simulink model "sensorMCU"  (Simulink 6.6)
settings: Solver=FixedStepDiscrete  StartTime=0.0  StopTime=10.0  FixedStep=0.01  RelTol=1e-3
InitFcn:
  | mcuInit
values from neighbouring files (symbols this model uses):
  gxGainrad = gxGain*pi/180    [mcuInit.m]
  gyGainrad = gyGain*pi/180    [mcuInit.m]
  gzGainrad = gzGain*pi/180    [mcuInit.m]
  T = 0.01    [initGPS.m]    (also in mcuInit.m)
undefined symbols (not defined in the file or in its folder): AccelParam, floatToBytes, gaind, gpsInit, gpsParse, gpsRead, gpsSeparate, gyTGain, hil_getEuler, hil_getGPSRead, hil_getRates, hil_getRawRead, hil_getVned, hil_getXYZ, hilRead, logData, loggerInit, MagParam, mzTGain, polesd, protParseDecode, protParserInit, shortToBytes, spiMasterInit, spiSend, stTGain, tmeanMz, tmeanSt, tmeanVl, u1, uartInit, uShortToBytes, vlTGain, y1, zerosd
libraries: dsPICdrivers x72, simulink x6, dspswit3 x1, dspsigops x1, xpclib x1, aerolibconvert2 x1
(part 2 of 3)

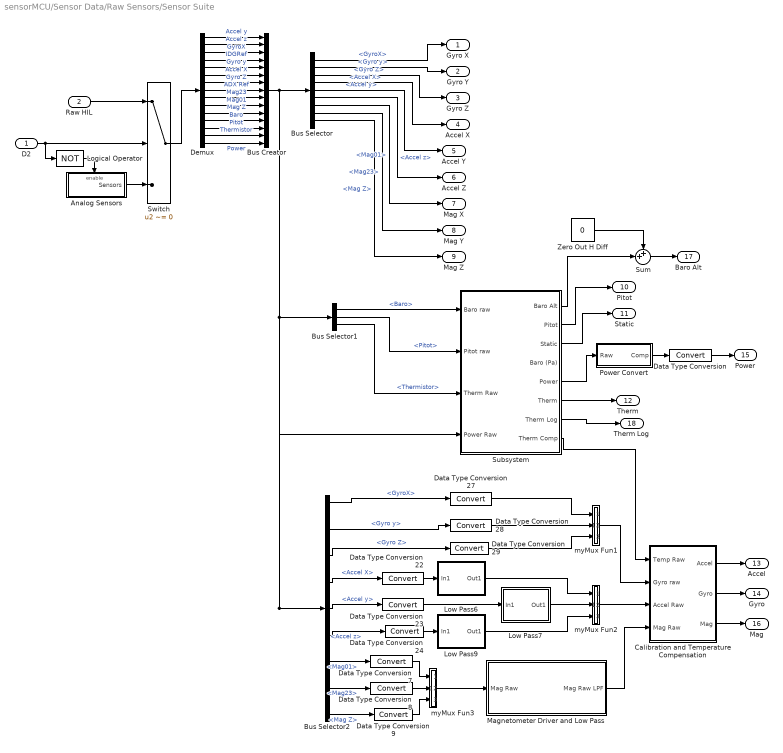
== system sensorMCU/Sensor Data/Raw Sensors/Sensor Suite ==
  D2 : Inport
  Raw HIL : Inport  Port=2
  Analog Sensors : Subsystem
  Bus Creator : BusCreator  Inputs=15
  Bus Selector : BusSelector  OutputSignals=GyroX,Gyro y,Gyro Z,Accel X,Accel y,Accel z,Mag01,Mag23,Mag Z
  Bus Selector1 : BusSelector  OutputSignals=Baro,Pitot,Thermistor
  Bus Selector2 : BusSelector  OutputSignals=GyroX,Gyro y,Gyro Z,Accel X,Accel y,Accel z,Mag01,Mag23,Mag Z
  Calibration and Temperature Compensation : Subsystem
  Data Type Conversion : DataTypeConversion  OutDataTypeMode=uint16
  Data Type Conversion{7..9,22..24,27..29} (9 alike) : DataTypeConversion  OutDataTypeMode=double
  Demux : Demux  Outputs=15
  Logical Operator : Logic  Operator=NOT  AllPortsSameDT=off  OutDataTypeMode=Boolean
  Low Pass6 : Subsystem  mask(DiscretizedZeroPole){Zeros=[], Poles=[-150], Gain=150, AbsTol=auto, SampleTime=T, method=tustin, Wc=1}
      mask prompts: Zeros "Zeros (enter in s-main:)"; Poles "Poles (enter in s-domain:)"; Gain "Gain (enter in s-domain:)"; AbsTol "Absolute tolerance:"; SampleTime "Sample time:"; Wc "Critical Frequency (Hz):"
      mask help: Continuous mask uses c2d to transform parameters onto the Discrete Zero-Pole block inside.
      mask init:
      | st=SampleTime;
      | if length(st)>1
      |     st=SampleTime(1);
      | end
      | if(st>0)
      |     [zerosd,polesd,gaind] = sldiscutil('disczpk', {st,method,Wc,Zeros,Poles,Gain});
      | end	
      | s = get_param(gcb,'maskvalues');
      | zeross = s{1};
      | poless = s{2};
      | gainss = s{3};
      | %zerosc = eval(zeross);
      | %polesc = eval(poless);
      | %gainsc = eval(gainss);
      | sldiscutil('initzpkmask', st);
      | if(st==0)
      | set_param([gcb '/Zero Pole'], 'AbsoluteTolerance', AbsTol);
      | end
      mask StyleString: edit,edit,edit,edit,edit,popup(zoh|foh|tustin|prewarp|matched),edit
      mask CallbackString: |||||hidecrit|
      mask Display:
      | droots(zeross,poless,gainss)
      | text( 0.5, 1.0, method, 'verticalAlignment','top')
  Low Pass7 : Subsystem  mask(DiscretizedZeroPole){Zeros=[], Poles=[-150], Gain=150, AbsTol=auto, SampleTime=T, method=tustin, Wc=1}
      mask prompts: Zeros "Zeros (enter in s-main:)"; Poles "Poles (enter in s-domain:)"; Gain "Gain (enter in s-domain:)"; AbsTol "Absolute tolerance:"; SampleTime "Sample time:"; Wc "Critical Frequency (Hz):"
      mask help: Continuous mask uses c2d to transform parameters onto the Discrete Zero-Pole block inside.
      mask init: same as sensorMCU/Sensor Data/Raw Sensors/Sensor Suite/Low Pass6
      mask StyleString: edit,edit,edit,edit,edit,popup(zoh|foh|tustin|prewarp|matched),edit
      mask CallbackString: |||||hidecrit|
      mask Display:
      | droots(zeross,poless,gainss)
      | text( 0.5, 1.0, method, 'verticalAlignment','top')
  Low Pass9 : Subsystem  mask(DiscretizedZeroPole){Zeros=[], Poles=[-150], Gain=150, AbsTol=auto, SampleTime=T, method=tustin, Wc=1}
      mask prompts: Zeros "Zeros (enter in s-main:)"; Poles "Poles (enter in s-domain:)"; Gain "Gain (enter in s-domain:)"; AbsTol "Absolute tolerance:"; SampleTime "Sample time:"; Wc "Critical Frequency (Hz):"
      mask help: Continuous mask uses c2d to transform parameters onto the Discrete Zero-Pole block inside.
      mask init: same as sensorMCU/Sensor Data/Raw Sensors/Sensor Suite/Low Pass6
      mask StyleString: edit,edit,edit,edit,edit,popup(zoh|foh|tustin|prewarp|matched),edit
      mask CallbackString: |||||hidecrit|
      mask Display:
      | droots(zeross,poless,gainss)
      | text( 0.5, 1.0, method, 'verticalAlignment','top')
  Magnetometer Driver and Low Pass : Subsystem
  Power Convert : Subsystem  mask{bias=0.02946, gains=0.003226}
      mask prompts: bias "Initial Bias"; gains "Initial Gains"
      mask help: Convert Analog readings to units
  Subsystem : Subsystem
  Sum : Sum  Inputs=++|
  Switch : Switch  Criteria=u2 ~= 0  SampleTime=0.01
  Zero Out H Diff : Constant  Value=0
  myMux Fun1 : Stateflow chart
  myMux Fun2 : Stateflow chart
  myMux Fun3 : Stateflow chart
  Gyro X : Outport
  Gyro Y : Outport  Port=2
  Gyro Z : Outport  Port=3
  Accel X : Outport  Port=4
  Accel Y : Outport  Port=5
  Accel Z : Outport  Port=6
  Mag X : Outport  Port=7
  Mag Y : Outport  Port=8
  Mag Z : Outport  Port=9
  Pitot : Outport  Port=10
  Static : Outport  Port=11
  Therm : Outport  Port=12
  Accel : Outport  Port=13
  Gyro : Outport  Port=14
  Power : Outport  Port=15
  Mag : Outport  Port=16
  Baro Alt : Outport  Port=17
  Therm Log : Outport  Port=18
  wires:
  Demux/1 -> Bus Creator/1  "Accel y"
  Demux/2 -> Bus Creator/2  "Accel z"
  Demux/3 -> Bus Creator/3  "GyroX"
  Demux/4 -> Bus Creator/4  "IDGRef"
  Demux/5 -> Bus Creator/5  "Gyro y"
  Demux/6 -> Bus Creator/6  "Accel X"
  Demux/7 -> Bus Creator/7  "Gyro Z"
  Demux/8 -> Bus Creator/8  "ADX Ref"
  Demux/9 -> Bus Creator/9  "Mag23"
  Demux/10 -> Bus Creator/10  "Mag01"
  Demux/11 -> Bus Creator/11  "Mag Z"
  Demux/12 -> Bus Creator/12  "Baro"
  Demux/13 -> Bus Creator/13  "Pitot"
  Demux/14 -> Bus Creator/14  "Thermistor"
  Demux/15 -> Bus Creator/15  "Power"
  Bus Creator/1 -> Bus Selector/1, Bus Selector1/1, Bus Selector2/1, Subsystem/4(Power Raw)
  Bus Selector1/1 -> Subsystem/1(Baro raw)  "<Baro>"
  Data Type Conversion27/1 -> myMux Fun1/1(u1)
  Data Type Conversion28/1 -> myMux Fun1/2(u2)
  Data Type Conversion29/1 -> myMux Fun1/3(u3)
  Low Pass6/1(Out1) -> myMux Fun2/1(u1)
  Low Pass7/1(Out1) -> myMux Fun2/2(u2)
  Data Type Conversion22/1 -> Low Pass6/1(In1)
  Data Type Conversion23/1 -> Low Pass7/1(In1)
  Data Type Conversion24/1 -> Low Pass9/1(In1)
  Low Pass9/1(Out1) -> myMux Fun2/3(u3)
  Bus Selector/1 -> Gyro X/1  "<GyroX>"
  Bus Selector/2 -> Gyro Y/1  "<Gyro y>"
  Bus Selector/3 -> Gyro Z/1  "<Gyro Z>"
  Bus Selector/4 -> Accel X/1  "<Accel X>"
  Bus Selector/5 -> Accel Y/1  "<Accel y>"
  Bus Selector/6 -> Accel Z/1  "<Accel z>"
  Bus Selector/7 -> Mag X/1  "<Mag01>"
  Bus Selector/8 -> Mag Y/1  "<Mag23>"
  Bus Selector/9 -> Mag Z/1  "<Mag Z>"
  Bus Selector2/1 -> Data Type Conversion27/1  "<GyroX>"
  Bus Selector2/2 -> Data Type Conversion28/1  "<Gyro y>"
  Bus Selector2/3 -> Data Type Conversion29/1  "<Gyro Z>"
  Bus Selector2/4 -> Data Type Conversion22/1  "<Accel X>"
  Bus Selector2/5 -> Data Type Conversion23/1  "<Accel y>"
  Bus Selector2/6 -> Data Type Conversion24/1  "<Accel z>"
  myMux Fun1/1(y) -> Calibration and Temperature Compensation/2(Gyro raw)
  myMux Fun2/1(y) -> Calibration and Temperature Compensation/3(Accel Raw)
  Bus Selector1/2 -> Subsystem/2(Pitot raw)  "<Pitot>"
  Bus Selector1/3 -> Subsystem/3(Therm Raw)  "<Thermistor>"
  Switch/1 -> Demux/1
  D2/1 -> Switch/2, Logical Operator/1
  Analog Sensors/1(Sensors) -> Switch/3
  Logical Operator/1 -> Analog Sensors/Enable
  Raw HIL/1 -> Switch/1
  Data Type Conversion7/1 -> myMux Fun3/1(u1)
  Data Type Conversion8/1 -> myMux Fun3/2(u2)
  Data Type Conversion9/1 -> myMux Fun3/3(u3)
  myMux Fun3/1(y) -> Magnetometer Driver and Low Pass/1(Mag Raw)
  Bus Selector2/7 -> Data Type Conversion7/1  "<Mag01>"
  Bus Selector2/8 -> Data Type Conversion8/1  "<Mag23>"
  Bus Selector2/9 -> Data Type Conversion9/1  "<Mag Z>"
  Calibration and Temperature Compensation/3(Mag) -> Mag/1
  Calibration and Temperature Compensation/1(Accel) -> Accel/1
  Calibration and Temperature Compensation/2(Gyro) -> Gyro/1
  Magnetometer Driver and Low Pass/1(Mag Raw LPF) -> Calibration and Temperature Compensation/4(Mag Raw)
  Subsystem/8(Therm Comp) -> Calibration and Temperature Compensation/1(Temp Raw)
  Subsystem/2(Pitot) -> Pitot/1
  Subsystem/3(Static) -> Static/1
  Subsystem/5(Power) -> Power Convert/1(Raw)
  Subsystem/6(Therm) -> Therm/1
  Subsystem/7(Therm Log) -> Therm Log/1
  Power Convert/1(Comp) -> Data Type Conversion/1
  Data Type Conversion/1 -> Power/1
  Sum/1 -> Baro Alt/1
  Subsystem/1(Baro Alt) -> Sum/2
  Zero Out H Diff/1 -> Sum/1

== system sensorMCU/Position-Attitude Filter/GPS parser/GPS Update/Detect Change ==
  Data : Inport
  Abs1 : Abs
  Difference1 : simulink/Discrete/Difference  SystemSampleTime=-1  ICPrevInput=0.0  OutDataType=sfix(16)  OutScaling=2^-10  DoSatur=off
  Saturation1 : Saturate  UpperLimit=1  LowerLimit=0
  change? : Outport
  wires:
  Difference1/1 -> Abs1/1
  Abs1/1 -> Saturation1/1
  Data/1 -> Difference1/1
  Saturation1/1 -> change?/1

== system sensorMCU/Position-Attitude Filter/GPS parser/GPS Update/Detect Change1 ==
  Data : Inport
  Abs1 : Abs
  Difference1 : simulink/Discrete/Difference  SystemSampleTime=-1  ICPrevInput=0.0  OutDataType=sfix(16)  OutScaling=2^-10  DoSatur=off
  Saturation1 : Saturate  UpperLimit=1  LowerLimit=0
  change? : Outport
  wires:
  Saturation1/1 -> change?/1
  Data/1 -> Difference1/1
  Abs1/1 -> Saturation1/1
  Difference1/1 -> Abs1/1

== system sensorMCU/Position-Attitude Filter/GPS parser/GPS Update/Detect Change2 ==
  Data : Inport
  Abs1 : Abs
  Difference1 : simulink/Discrete/Difference  SystemSampleTime=-1  ICPrevInput=0.0  OutDataType=sfix(16)  OutScaling=2^-10  DoSatur=off
  Saturation1 : Saturate  UpperLimit=1  LowerLimit=0
  change? : Outport
  wires:
  Difference1/1 -> Abs1/1
  Abs1/1 -> Saturation1/1
  Data/1 -> Difference1/1
  Saturation1/1 -> change?/1

== system sensorMCU/Position-Attitude Filter/GPS parser/Geod2LTP2/ECEF2LTP (UEN) ==
  ECEF coordinates : Inport
  "Long, Lat" : Inport  Port=2
  Deg2R : Gain  Gain=pi/180  SaturateOnIntegerOverflow=on
  Demux3 : Demux  Outputs=2
  From Body to Universal1 : Subsystem
  Product1 : Product  Multiplication=Matrix(*)  SaturateOnIntegerOverflow=on  InputSameDT=on
  Out : Outport
  wires:
  "Long, Lat"/1 -> Deg2R/1
  Product1/1 -> Out/1
  Demux3/2 -> From Body to Universal1/2(lat)
  Demux3/1 -> From Body to Universal1/1(long)
  Deg2R/1 -> Demux3/1
  ECEF coordinates/1 -> Product1/2
  From Body to Universal1/1(DCM) -> Product1/1

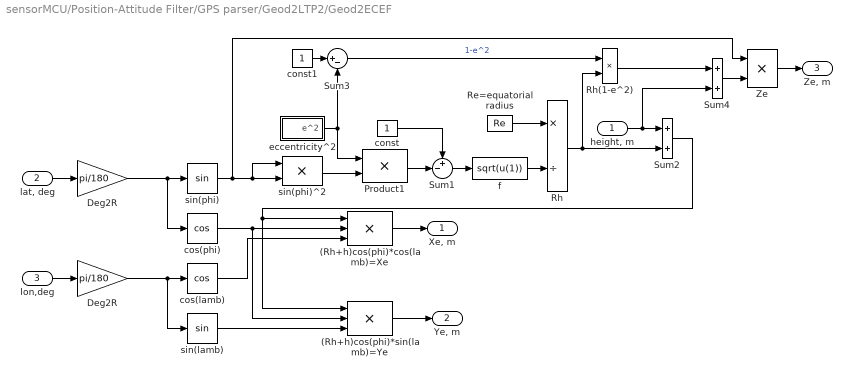
== system sensorMCU/Position-Attitude Filter/GPS parser/Geod2LTP2/Geod2ECEF ==
  "height, m" : Inport
  "lat, deg" : Inport  Port=2
  lon,deg : Inport  Port=3
  (Rh+h)cos(phi)*cos(lamb)=Xe : Product  Inputs=3  SaturateOnIntegerOverflow=on  InputSameDT=on
  (Rh+h)cos(phi)*sin(lamb)=Ye : Product  Inputs=3  SaturateOnIntegerOverflow=on  InputSameDT=on
  Deg2R : Gain  Gain=pi/180  SaturateOnIntegerOverflow=on
  "Deg2R " : Gain  Gain=pi/180  SaturateOnIntegerOverflow=on
  Product1 : Product  SaturateOnIntegerOverflow=on  InputSameDT=on
  Re=equatorial radius : Constant  Value=Re
  Rh : Product  Inputs=*/  SaturateOnIntegerOverflow=on  InputSameDT=on
  Rh(1-e^2) : Product  SaturateOnIntegerOverflow=on  InputSameDT=on
  Sum1 : Sum  Inputs=+-|  SaturateOnIntegerOverflow=on  InputSameDT=on
  Sum2 : Sum  SaturateOnIntegerOverflow=on  InputSameDT=on
      settings: AttributesFormatString=Rh+h
  Sum3 : Sum  Inputs=|+-  SaturateOnIntegerOverflow=on  InputSameDT=on
  Sum4 : Sum  SaturateOnIntegerOverflow=on  InputSameDT=on
      settings: AttributesFormatString=(1-e^2)Rh+h
  Ze : Product  SaturateOnIntegerOverflow=on  InputSameDT=on
  const : Constant
  const1 : Constant
  cos(lamb) : Trigonometry  Operator=cos
  cos(phi) : Trigonometry  Operator=cos
  eccentricity^2 : Subsystem
  f : Fcn  Expr=sqrt(u(1))
  sin(lamb) : Trigonometry
  sin(phi) : Trigonometry
  sin(phi)^2 : Product  SaturateOnIntegerOverflow=on  InputSameDT=on
  "Xe, m " : Outport
  "Ye, m " : Outport  Port=2
  "Ze, m " : Outport  Port=3
  wires:
  "lat, deg"/1 -> Deg2R/1
  sin(phi)/1 -> sin(phi)^2/1, sin(phi)^2/2, Ze/1
  f/1 -> Rh/2
  Re=equatorial radius/1 -> Rh/1
  Rh/1 -> Sum2/2, Rh(1-e^2)/2
  Product1/1 -> Sum1/2
  Sum1/1 -> f/1
  const/1 -> Sum1/1
  "height, m"/1 -> Sum4/2, Sum2/1
  eccentricity^2/1(e^2) -> Product1/1, Sum3/2
  sin(phi)^2/1 -> Product1/2
  const1/1 -> Sum3/1
  Sum3/1 -> Rh(1-e^2)/1  "1-e^2"
  Rh(1-e^2)/1 -> Sum4/1
  Sum4/1 -> Ze/2
  lon,deg/1 -> "Deg2R "/1
  cos(phi)/1 -> (Rh+h)cos(phi)*cos(lamb)=Xe/2, (Rh+h)cos(phi)*sin(lamb)=Ye/2
  cos(lamb)/1 -> (Rh+h)cos(phi)*cos(lamb)=Xe/3
  sin(lamb)/1 -> (Rh+h)cos(phi)*sin(lamb)=Ye/3
  Ze/1 -> "Ze, m "/1
  Deg2R/1 -> cos(phi)/1, sin(phi)/1
  "Deg2R "/1 -> cos(lamb)/1, sin(lamb)/1
  Sum2/1 -> (Rh+h)cos(phi)*sin(lamb)=Ye/1, (Rh+h)cos(phi)*cos(lamb)=Xe/1
  (Rh+h)cos(phi)*cos(lamb)=Xe/1 -> "Xe, m "/1
  (Rh+h)cos(phi)*sin(lamb)=Ye/1 -> "Ye, m "/1

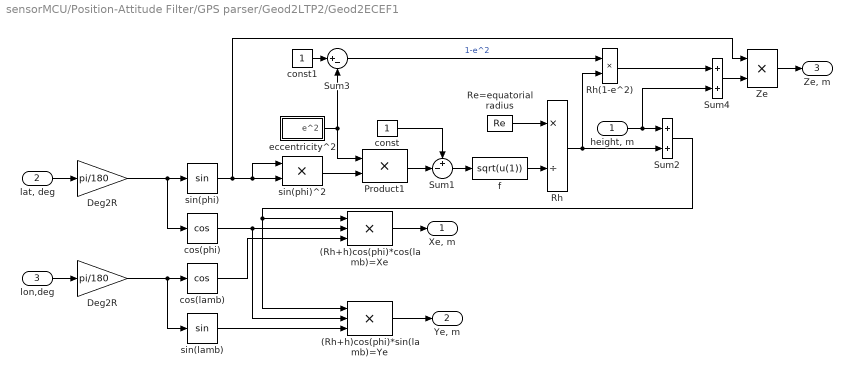
== system sensorMCU/Position-Attitude Filter/GPS parser/Geod2LTP2/Geod2ECEF1 ==
  "height, m" : Inport
  "lat, deg" : Inport  Port=2
  lon,deg : Inport  Port=3
  (Rh+h)cos(phi)*cos(lamb)=Xe : Product  Inputs=3  SaturateOnIntegerOverflow=on  InputSameDT=on
  (Rh+h)cos(phi)*sin(lamb)=Ye : Product  Inputs=3  SaturateOnIntegerOverflow=on  InputSameDT=on
  Deg2R : Gain  Gain=pi/180  SaturateOnIntegerOverflow=on
  "Deg2R " : Gain  Gain=pi/180  SaturateOnIntegerOverflow=on
  Product1 : Product  SaturateOnIntegerOverflow=on  InputSameDT=on
  Re=equatorial radius : Constant  Value=Re
  Rh : Product  Inputs=*/  SaturateOnIntegerOverflow=on  InputSameDT=on
  Rh(1-e^2) : Product  SaturateOnIntegerOverflow=on  InputSameDT=on
  Sum1 : Sum  Inputs=+-|  SaturateOnIntegerOverflow=on  InputSameDT=on
  Sum2 : Sum  SaturateOnIntegerOverflow=on  InputSameDT=on
      settings: AttributesFormatString=Rh+h
  Sum3 : Sum  Inputs=|+-  SaturateOnIntegerOverflow=on  InputSameDT=on
  Sum4 : Sum  SaturateOnIntegerOverflow=on  InputSameDT=on
      settings: AttributesFormatString=(1-e^2)Rh+h
  Ze : Product  SaturateOnIntegerOverflow=on  InputSameDT=on
  const : Constant
  const1 : Constant
  cos(lamb) : Trigonometry  Operator=cos
  cos(phi) : Trigonometry  Operator=cos
  eccentricity^2 : Subsystem
  f : Fcn  Expr=sqrt(u(1))
  sin(lamb) : Trigonometry
  sin(phi) : Trigonometry
  sin(phi)^2 : Product  SaturateOnIntegerOverflow=on  InputSameDT=on
  "Xe, m " : Outport
  "Ye, m " : Outport  Port=2
  "Ze, m " : Outport  Port=3
  wires:
  (Rh+h)cos(phi)*sin(lamb)=Ye/1 -> "Ye, m "/1
  (Rh+h)cos(phi)*cos(lamb)=Xe/1 -> "Xe, m "/1
  Sum2/1 -> (Rh+h)cos(phi)*cos(lamb)=Xe/1, (Rh+h)cos(phi)*sin(lamb)=Ye/1
  "Deg2R "/1 -> sin(lamb)/1, cos(lamb)/1
  Deg2R/1 -> sin(phi)/1, cos(phi)/1
  Ze/1 -> "Ze, m "/1
  sin(lamb)/1 -> (Rh+h)cos(phi)*sin(lamb)=Ye/3
  cos(lamb)/1 -> (Rh+h)cos(phi)*cos(lamb)=Xe/3
  cos(phi)/1 -> (Rh+h)cos(phi)*sin(lamb)=Ye/2, (Rh+h)cos(phi)*cos(lamb)=Xe/2
  lon,deg/1 -> "Deg2R "/1
  Sum4/1 -> Ze/2
  Rh(1-e^2)/1 -> Sum4/1
  Sum3/1 -> Rh(1-e^2)/1  "1-e^2"
  const1/1 -> Sum3/1
  sin(phi)^2/1 -> Product1/2
  eccentricity^2/1(e^2) -> Sum3/2, Product1/1
  "height, m"/1 -> Sum2/1, Sum4/2
  const/1 -> Sum1/1
  Sum1/1 -> f/1
  Product1/1 -> Sum1/2
  Rh/1 -> Rh(1-e^2)/2, Sum2/2
  Re=equatorial radius/1 -> Rh/1
  f/1 -> Rh/2
  sin(phi)/1 -> Ze/1, sin(phi)^2/2, sin(phi)^2/1
  "lat, deg"/1 -> Deg2R/1

== system sensorMCU/Sensor Data/Raw Sensors/Sensor Suite/Analog Sensors ==
  Enable : EnablePort
  ADC Input : dsPICdrivers/Peripheral I//O/ADC Input  Tag=dsPIC_ADC  Priority=5  ADC_TYPE=12 bits  ADC_MODE=Continuous sampling & get last channel value  NbrSampleStep=1  VoltRefpopup="AVdd  -  AVss"  OutFormatBitspopup=0000 dddd dddd dddd : Integer  InterruptPriority=6  ANCHANNELS=[0 1 3 4 5 6 7 8 9 10 11 12 13 15 16]  MaxName=ANmax = 4096  Rin=1e2  ADCS=53  SAMC=1  Temperature=25  DMAChannel=1  SampleTime=.01  Status="OK  |  Tsmp=6.750e-007 |  T/Channel=1.012e-005 |  Tall=1.519e-004"
  Mux : Mux  Inputs=15
  Sensors : Outport
  wires:
  ADC Input/1 -> Mux/1
  ADC Input/2 -> Mux/2
  ADC Input/3 -> Mux/3
  ADC Input/4 -> Mux/4
  ADC Input/5 -> Mux/5
  ADC Input/6 -> Mux/6
  ADC Input/7 -> Mux/7
  ADC Input/8 -> Mux/8
  ADC Input/9 -> Mux/9
  ADC Input/10 -> Mux/10
  ADC Input/11 -> Mux/11
  ADC Input/12 -> Mux/12
  ADC Input/13 -> Mux/13
  ADC Input/14 -> Mux/14
  ADC Input/15 -> Mux/15
  Mux/1 -> Sensors/1

== system sensorMCU/Sensor Data/Raw Sensors/Sensor Suite/Calibration and Temperature Compensation ==
  Temp Raw : Inport
  Gyro raw : Inport  Port=2
  Accel Raw : Inport  Port=3
  Mag Raw : Inport  Port=4
  AccelConvert : Subsystem  mask{bias=[AccelParam.xo AccelParam.yo AccelParam.zo], gains=[-AccelParam.a AccelParam.b  -AccelParam.c]}
      mask prompts: bias "Initial Bias"; gains "Initial Gains"
      mask help: Convert Analog readings to units
  Divide : Product  OutScaling=2^-10
  Enables/Disables the Computation of  initial Biases and Temps : Stateflow chart
  Gyro Gains : Constant  Value=[-gxGainrad gyGainrad gzGainrad]
  Gyro Temp  Compensation : Subsystem  mask{alpha=[0 gyTGain 0]}
      mask prompts: alpha "Gyro Tempearature Coeficientt"
      mask help: Temperature Compensate Gyro Measurement
  Initial Bias and Temp : Subsystem  TreatAsAtomicUnit=on
  Mag Convert : Subsystem  mask{bias=[MagParam.xo MagParam.yo MagParam.zo], gains=[MagParam.a MagParam.b  MagParam.c]}
      mask prompts: bias "Initial Bias"; gains "Initial Gains"
      mask help: Convert Analog readings to units
  Mag Temp  Compensation : Subsystem  mask{alpha=[0 0 mzTGain], tempMean=[0 0 tmeanMz]}
      mask prompts: alpha "Tempearature Coeficientt"; tempMean "Calibration Mean Temperature"
      mask help: Temperature Compensate Gyro Measurement
  Accel : Outport
  Gyro : Outport  Port=2
  Mag : Outport  Port=3
  wires:
  AccelConvert/1(Comp) -> Accel/1
  Accel Raw/1 -> AccelConvert/1(Raw)
  Enables/Disables the Computation of  initial Biases and Temps/1(tOut) -> Initial Bias and Temp/Enable
  Temp Raw/1 -> Initial Bias and Temp/1(Temp Raw), Gyro Temp  Compensation/4(Temp Raw), Mag Temp  Compensation/1(Temp Raw)
  Gyro raw/1 -> Initial Bias and Temp/2(Gyro Raw), Gyro Temp  Compensation/3(Raw)
  Initial Bias and Temp/2(Gyro Ini Bias) -> Gyro Temp  Compensation/2(Bias Ini)
  Initial Bias and Temp/1(Temp Ini) -> Gyro Temp  Compensation/1(Temp Ini)
  Gyro Temp  Compensation/1(Comp) -> Divide/1
  Gyro Gains/1 -> Divide/2
  Divide/1 -> Gyro/1
  Mag Raw/1 -> Mag Temp  Compensation/2(Raw)
  Mag Convert/1(Comp) -> Mag/1
  Mag Temp  Compensation/1(Comp) -> Mag Convert/1(Raw)

== system sensorMCU/Sensor Data/Raw Sensors/Sensor Suite/Low Pass6 ==
  In1 : Inport
  Discrete Zero-Pole : DiscreteZeroPole  Zeros=zerosd  Poles=polesd  Gain=gaind  SampleTime=SampleTime
  Out1 : Outport
  wires:
  In1/1 -> Discrete Zero-Pole/1
  Discrete Zero-Pole/1 -> Out1/1

== system sensorMCU/Sensor Data/Raw Sensors/Sensor Suite/Low Pass7 ==
  In1 : Inport
  Discrete Zero-Pole : DiscreteZeroPole  Zeros=zerosd  Poles=polesd  Gain=gaind  SampleTime=SampleTime
  Out1 : Outport
  wires:
  Discrete Zero-Pole/1 -> Out1/1
  In1/1 -> Discrete Zero-Pole/1

== system sensorMCU/Sensor Data/Raw Sensors/Sensor Suite/Low Pass9 ==
  In1 : Inport
  Discrete Zero-Pole : DiscreteZeroPole  Zeros=zerosd  Poles=polesd  Gain=gaind  SampleTime=SampleTime
  Out1 : Outport
  wires:
  Discrete Zero-Pole/1 -> Out1/1
  In1/1 -> Discrete Zero-Pole/1

== system sensorMCU/Sensor Data/Raw Sensors/Sensor Suite/Magnetometer Driver and Low Pass ==
  Mag Raw : Inport
  Demux1 : Demux  Outputs=3
  Low Pass3 : Subsystem  mask(DiscretizedZeroPole){Zeros=[], Poles=[-150], Gain=150, AbsTol=auto, SampleTime=T, method=tustin, Wc=1}
      mask prompts: Zeros "Zeros (enter in s-main:)"; Poles "Poles (enter in s-domain:)"; Gain "Gain (enter in s-domain:)"; AbsTol "Absolute tolerance:"; SampleTime "Sample time:"; Wc "Critical Frequency (Hz):"
      mask help: Continuous mask uses c2d to transform parameters onto the Discrete Zero-Pole block inside.
      mask init: same as sensorMCU/Sensor Data/Raw Sensors/Sensor Suite/Low Pass6
      mask StyleString: edit,edit,edit,edit,edit,popup(zoh|foh|tustin|prewarp|matched),edit
      mask CallbackString: |||||hidecrit|
      mask Display:
      | droots(zeross,poless,gainss)
      | text( 0.5, 1.0, method, 'verticalAlignment','top')
  Low Pass4 : Subsystem  mask(DiscretizedZeroPole){Zeros=[], Poles=[-150], Gain=150, AbsTol=auto, SampleTime=T, method=tustin, Wc=1}
      mask prompts: Zeros "Zeros (enter in s-main:)"; Poles "Poles (enter in s-domain:)"; Gain "Gain (enter in s-domain:)"; AbsTol "Absolute tolerance:"; SampleTime "Sample time:"; Wc "Critical Frequency (Hz):"
      mask help: Continuous mask uses c2d to transform parameters onto the Discrete Zero-Pole block inside.
      mask init: same as sensorMCU/Sensor Data/Raw Sensors/Sensor Suite/Low Pass6
      mask StyleString: edit,edit,edit,edit,edit,popup(zoh|foh|tustin|prewarp|matched),edit
      mask CallbackString: |||||hidecrit|
      mask Display:
      | droots(zeross,poless,gainss)
      | text( 0.5, 1.0, method, 'verticalAlignment','top')
  Low Pass5 : Subsystem  mask(DiscretizedZeroPole){Zeros=[], Poles=[-150], Gain=150, AbsTol=auto, SampleTime=T, method=tustin, Wc=1}
      mask prompts: Zeros "Zeros (enter in s-main:)"; Poles "Poles (enter in s-domain:)"; Gain "Gain (enter in s-domain:)"; AbsTol "Absolute tolerance:"; SampleTime "Sample time:"; Wc "Critical Frequency (Hz):"
      mask help: Continuous mask uses c2d to transform parameters onto the Discrete Zero-Pole block inside.
      mask init: same as sensorMCU/Sensor Data/Raw Sensors/Sensor Suite/Low Pass6
      mask StyleString: edit,edit,edit,edit,edit,popup(zoh|foh|tustin|prewarp|matched),edit
      mask CallbackString: |||||hidecrit|
      mask Display:
      | droots(zeross,poless,gainss)
      | text( 0.5, 1.0, method, 'verticalAlignment','top')
  Magnetometer Driver : Stateflow chart
  myMux Fun1 : Stateflow chart
  Mag Raw LPF : Outport
  wires:
  Magnetometer Driver/1(mag_k) -> Demux1/1
  Demux1/1 -> Low Pass3/1(In1)
  Demux1/2 -> Low Pass4/1(In1)
  Demux1/3 -> Low Pass5/1(In1)
  Mag Raw/1 -> Magnetometer Driver/1(M_in)
  myMux Fun1/1(y) -> Mag Raw LPF/1
  Low Pass3/1(Out1) -> myMux Fun1/1(u1)
  Low Pass4/1(Out1) -> myMux Fun1/2(u2)
  Low Pass5/1(Out1) -> myMux Fun1/3(u3)

== system sensorMCU/Sensor Data/Raw Sensors/Sensor Suite/Power Convert ==
  Raw : Inport
  Bias : Constant  Value=bias
  Divide : Product  OutScaling=2^-10
  Gain : Gain  Gain=1000
  Gains : Constant  Value=gains
  Sum : Sum  Inputs=|++
  Comp : Outport
  wires:
  Bias/1 -> Sum/2
  Raw/1 -> Divide/2
  Gains/1 -> Divide/1
  Divide/1 -> Sum/1
  Sum/1 -> Gain/1
  Gain/1 -> Comp/1

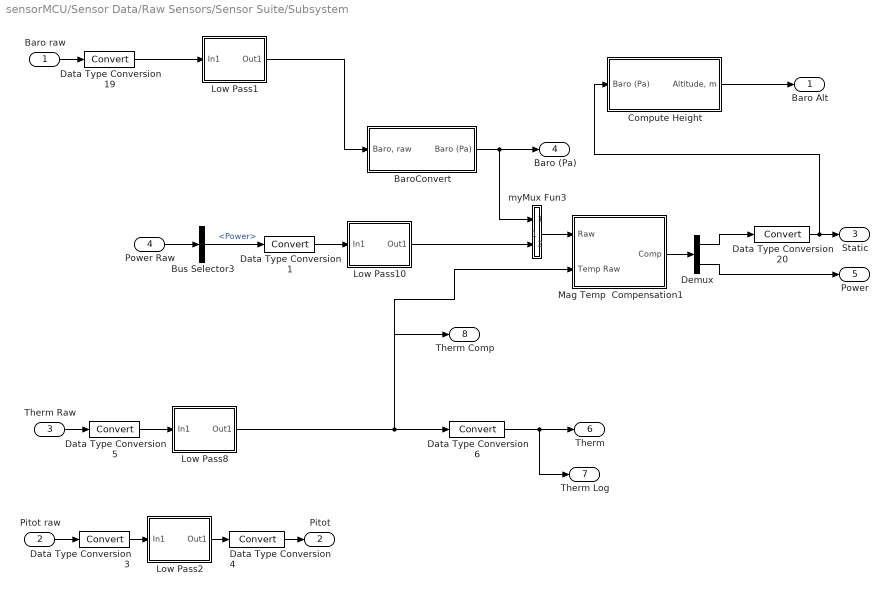
== system sensorMCU/Sensor Data/Raw Sensors/Sensor Suite/Subsystem ==
  Baro raw : Inport
  Pitot raw : Inport  Port=2
  Therm Raw : Inport  Port=3
  Power Raw : Inport  Port=4
  BaroConvert : Subsystem  mask{bias=4664.3, gains=28.508}
      mask prompts: bias "Initial Bias"; gains "Initial Gains"
      mask help: Convert Analog readings to units
  Bus Selector3 : BusSelector  OutputSignals=Power
  Compute Height : Subsystem  mask{bGain=28.508, bBias=4664.3, basePressure=98192.64, baseTemp=288.215, LapseRate=-0.00198122, baseHeight=225}
      mask prompts: bGain "Barometer Gain"; bBias "Barometer Bias"; basePressure "Base Station Pressure (Pa)"; baseTemp "Base Station Temperature (K)"; LapseRate "Lapse Rate (C/ft)"; baseHeight "Base Station Known Height (m)"
      mask help:
      | Produces Altitude in meters from Raw Baro Altimeter. Altitude is valid from MSL to 6000 ft.
      |
      | The method implemented here was developed by Ren Curry
  Data Type Conversion{1,3,5,19} (4 alike) : DataTypeConversion  OutDataTypeMode=double
  Data Type Conversion20 : DataTypeConversion  OutDataTypeMode=single
  Data Type Conversion4 : DataTypeConversion  OutDataTypeMode=single
  Data Type Conversion6 : DataTypeConversion  OutDataTypeMode=int16
  Demux : Demux  Outputs=2
  Low Pass1 : Subsystem  mask(DiscretizedZeroPole){Zeros=[], Poles=[-5], Gain=5, AbsTol=auto, SampleTime=T, method=tustin, Wc=1}
      mask prompts: Zeros "Zeros (enter in s-main:)"; Poles "Poles (enter in s-domain:)"; Gain "Gain (enter in s-domain:)"; AbsTol "Absolute tolerance:"; SampleTime "Sample time:"; Wc "Critical Frequency (Hz):"
      mask help: Continuous mask uses c2d to transform parameters onto the Discrete Zero-Pole block inside.
      mask init: same as sensorMCU/Sensor Data/Raw Sensors/Sensor Suite/Low Pass6
      mask StyleString: edit,edit,edit,edit,edit,popup(zoh|foh|tustin|prewarp|matched),edit
      mask CallbackString: |||||hidecrit|
      mask Display:
      | droots(zeross,poless,gainss)
      | text( 0.5, 1.0, method, 'verticalAlignment','top')
  Low Pass10 : Subsystem  mask(DiscretizedZeroPole){Zeros=[], Poles=[-150], Gain=150, AbsTol=auto, SampleTime=T, method=tustin, Wc=1}
      mask prompts: Zeros "Zeros (enter in s-main:)"; Poles "Poles (enter in s-domain:)"; Gain "Gain (enter in s-domain:)"; AbsTol "Absolute tolerance:"; SampleTime "Sample time:"; Wc "Critical Frequency (Hz):"
      mask help: Continuous mask uses c2d to transform parameters onto the Discrete Zero-Pole block inside.
      mask init: same as sensorMCU/Sensor Data/Raw Sensors/Sensor Suite/Low Pass6
      mask StyleString: edit,edit,edit,edit,edit,popup(zoh|foh|tustin|prewarp|matched),edit
      mask CallbackString: |||||hidecrit|
      mask Display:
      | droots(zeross,poless,gainss)
      | text( 0.5, 1.0, method, 'verticalAlignment','top')
  Low Pass2 : Subsystem  mask(DiscretizedZeroPole){Zeros=[], Poles=[-30], Gain=30, AbsTol=auto, SampleTime=T, method=tustin, Wc=1}
      mask prompts: Zeros "Zeros (enter in s-main:)"; Poles "Poles (enter in s-domain:)"; Gain "Gain (enter in s-domain:)"; AbsTol "Absolute tolerance:"; SampleTime "Sample time:"; Wc "Critical Frequency (Hz):"
      mask help: Continuous mask uses c2d to transform parameters onto the Discrete Zero-Pole block inside.
      mask init: same as sensorMCU/Sensor Data/Raw Sensors/Sensor Suite/Low Pass6
      mask StyleString: edit,edit,edit,edit,edit,popup(zoh|foh|tustin|prewarp|matched),edit
      mask CallbackString: |||||hidecrit|
      mask Display:
      | droots(zeross,poless,gainss)
      | text( 0.5, 1.0, method, 'verticalAlignment','top')
  Low Pass8 : Subsystem  mask(DiscretizedZeroPole){Zeros=[], Poles=[-3], Gain=3, AbsTol=auto, SampleTime=T, method=tustin, Wc=1}
      mask prompts: Zeros "Zeros (enter in s-main:)"; Poles "Poles (enter in s-domain:)"; Gain "Gain (enter in s-domain:)"; AbsTol "Absolute tolerance:"; SampleTime "Sample time:"; Wc "Critical Frequency (Hz):"
      mask help: Continuous mask uses c2d to transform parameters onto the Discrete Zero-Pole block inside.
      mask init: same as sensorMCU/Sensor Data/Raw Sensors/Sensor Suite/Low Pass6
      mask StyleString: edit,edit,edit,edit,edit,popup(zoh|foh|tustin|prewarp|matched),edit
      mask CallbackString: |||||hidecrit|
      mask Display:
      | droots(zeross,poless,gainss)
      | text( 0.5, 1.0, method, 'verticalAlignment','top')
  Mag Temp  Compensation1 : Subsystem  mask{alpha=[stTGain vlTGain], tempMean=[tmeanSt tmeanVl]}
      mask prompts: alpha "Tempearature Coeficientt"; tempMean "Calibration Temperature Mean"
      mask help: Temperature Compensate Gyro Measurement
  myMux Fun3 : Stateflow chart
  Baro Alt : Outport
  Pitot : Outport  Port=2
  Static : Outport  Port=3
  Baro (Pa) : Outport  Port=4
  Power : Outport  Port=5
  Therm : Outport  Port=6
  Therm Log : Outport  Port=7
  Therm Comp : Outport  Port=8
  wires:
  Data Type Conversion19/1 -> Low Pass1/1(In1)
  Low Pass1/1(Out1) -> BaroConvert/1("Baro, raw")
  Data Type Conversion1/1 -> Low Pass10/1(In1)
  Bus Selector3/1 -> Data Type Conversion1/1  "<Power>"
  Data Type Conversion3/1 -> Low Pass2/1(In1)
  Low Pass2/1(Out1) -> Data Type Conversion4/1
  Data Type Conversion5/1 -> Low Pass8/1(In1)
  Low Pass8/1(Out1) -> Data Type Conversion6/1, Therm Comp/1, Mag Temp  Compensation1/2(Temp Raw)
  Data Type Conversion6/1 -> Therm/1, Therm Log/1
  Data Type Conversion4/1 -> Pitot/1
  Compute Height/1("Altitude, m") -> Baro Alt/1
  Data Type Conversion20/1 -> Static/1, Compute Height/1(Baro (Pa))
  Power Raw/1 -> Bus Selector3/1
  Baro raw/1 -> Data Type Conversion19/1
  Pitot raw/1 -> Data Type Conversion3/1
  BaroConvert/1(Baro (Pa)) -> Baro (Pa)/1, myMux Fun3/1(u1)
  Therm Raw/1 -> Data Type Conversion5/1
  Mag Temp  Compensation1/1(Comp) -> Demux/1
  Demux/1 -> Data Type Conversion20/1
  Demux/2 -> Power/1
  myMux Fun3/1(y) -> Mag Temp  Compensation1/1(Raw)
  Low Pass10/1(Out1) -> myMux Fun3/2(u2)

== system sensorMCU/Position-Attitude Filter/GPS parser/Geod2LTP2/ECEF2LTP (UEN)/From Body to Universal1 ==
  long : Inport
  lat : Inport  Port=2
  Mux : Mux  Inputs=2
  Reshape 9x1->3x1 : S-Function  FunctionName=sreshape  Parameters=OutputDimensionality, OutputDimensions  mask(Reshape){OutputDimensionality=Customize, OutputDimensions=[3,3]}
      mask prompts: OutputDimensionality "Output dimensionality:"; OutputDimensions "Output dimensions:"
      mask help:
      | Change the dimensions of a vector or matrix input signal. Output
      |  - a one-dimensional array (vector),
      |  - a column vector (Mx1 matrix),
      |  - a row vector (1xN matrix), or
      |  - a matrix or vector with specified dimensions, e.g., [M, N] or [W].
      mask init:
      | s = reshapemask(gcb,'init');
      mask StyleString: popup(1-D array|Column vector|Row vector|Customize),edit
      mask CallbackString: reshapemask(gcb,'cbDimensionality')|
      mask Display: disp('Reshape')
  Rotation Matrix from Long//Lat : Subsystem
      mask Type: Vector Transformation
      mask Description: Vector Transformation
      mask Display: disp('axis')
  DCM : Outport
  wires:
  lat/1 -> Mux/2
  long/1 -> Mux/1
  Mux/1 -> Rotation Matrix from Long//Lat/1(long lat)
  Rotation Matrix from Long//Lat/1(DCM) -> Reshape 9x1->3x1/1
  Reshape 9x1->3x1/1 -> DCM/1

== system sensorMCU/Position-Attitude Filter/GPS parser/Geod2LTP2/Geod2ECEF/eccentricity^2 ==
  " " : Product  SaturateOnIntegerOverflow=on  InputSameDT=on
  Re=equatorial radius1 : Constant  Value=Re
  Rp=polar radius : Constant  Value=Rp
  Sum5 : Sum  Inputs=|+-  SaturateOnIntegerOverflow=on  InputSameDT=on
  const2 : Constant
  e^1 : Product  Inputs=*/  SaturateOnIntegerOverflow=on  InputSameDT=on
  e^2 : Outport
  wires:
  Re=equatorial radius1/1 -> e^1/2
  Rp=polar radius/1 -> e^1/1
  const2/1 -> Sum5/1
  e^1/1 -> " "/2, " "/1
  " "/1 -> Sum5/2
  Sum5/1 -> e^2/1

== system sensorMCU/Position-Attitude Filter/GPS parser/Geod2LTP2/Geod2ECEF1/eccentricity^2 ==
  " " : Product  SaturateOnIntegerOverflow=on  InputSameDT=on
  Re=equatorial radius1 : Constant  Value=Re
  Rp=polar radius : Constant  Value=Rp
  Sum5 : Sum  Inputs=|+-  SaturateOnIntegerOverflow=on  InputSameDT=on
  const2 : Constant
  e^1 : Product  Inputs=*/  SaturateOnIntegerOverflow=on  InputSameDT=on
  e^2 : Outport
  wires:
  Sum5/1 -> e^2/1
  " "/1 -> Sum5/2
  e^1/1 -> " "/1, " "/2
  const2/1 -> Sum5/1
  Rp=polar radius/1 -> e^1/1
  Re=equatorial radius1/1 -> e^1/2

== system sensorMCU/Sensor Data/Raw Sensors/Sensor Suite/Calibration and Temperature Compensation/AccelConvert ==
  Raw : Inport
  Bias : Constant  Value=bias
  Divide : Product  Inputs=/*  OutScaling=2^-10
  Gains : Constant  Value=gains
  Sum : Sum  Inputs=|+-
  Comp : Outport
  wires:
  Raw/1 -> Sum/1
  Divide/1 -> Comp/1
  Sum/1 -> Divide/2
  Gains/1 -> Divide/1
  Bias/1 -> Sum/2

== system sensorMCU/Sensor Data/Raw Sensors/Sensor Suite/Calibration and Temperature Compensation/Gyro Temp  Compensation ==
  Temp Ini : Inport
  Bias Ini : Inport  Port=2
  Raw : Inport  Port=3
  Temp Raw : Inport  Port=4
  Divide1 : Product  OutScaling=2^-10
  Sum : Sum  Inputs=|+-
  Sum1 : Sum  Inputs=|+-
  Sum2 : Sum  Inputs=|+-
  gains : Constant  Value=alpha
  Comp : Outport
  wires:
  Sum/1 -> Sum2/1
  Raw/1 -> Sum/1
  Bias Ini/1 -> Sum/2
  Temp Ini/1 -> Sum1/2
  Temp Raw/1 -> Sum1/1
  Sum1/1 -> Divide1/2
  gains/1 -> Divide1/1
  Divide1/1 -> Sum2/2
  Sum2/1 -> Comp/1

== system sensorMCU/Sensor Data/Raw Sensors/Sensor Suite/Calibration and Temperature Compensation/Initial Bias and Temp ==
  Temp Raw : Inport
  Gyro Raw : Inport  Port=2
  Enable : EnablePort
  Demux : Demux  Outputs=3
  Low Pass1 : Subsystem  mask(DiscretizedZeroPole){Zeros=[], Poles=[-3], Gain=3, AbsTol=auto, SampleTime=T, method=tustin, Wc=1}
      mask prompts: Zeros "Zeros (enter in s-main:)"; Poles "Poles (enter in s-domain:)"; Gain "Gain (enter in s-domain:)"; AbsTol "Absolute tolerance:"; SampleTime "Sample time:"; Wc "Critical Frequency (Hz):"
      mask help: Continuous mask uses c2d to transform parameters onto the Discrete Zero-Pole block inside.
      mask init: same as sensorMCU/Sensor Data/Raw Sensors/Sensor Suite/Low Pass6
      mask StyleString: edit,edit,edit,edit,edit,popup(zoh|foh|tustin|prewarp|matched),edit
      mask CallbackString: |||||hidecrit|
      mask Display:
      | droots(zeross,poless,gainss)
      | text( 0.5, 1.0, method, 'verticalAlignment','top')
  Low Pass2 : Subsystem  mask(DiscretizedZeroPole){Zeros=[], Poles=[-3], Gain=3, AbsTol=auto, SampleTime=T, method=tustin, Wc=1}
      mask prompts: Zeros "Zeros (enter in s-main:)"; Poles "Poles (enter in s-domain:)"; Gain "Gain (enter in s-domain:)"; AbsTol "Absolute tolerance:"; SampleTime "Sample time:"; Wc "Critical Frequency (Hz):"
      mask help: Continuous mask uses c2d to transform parameters onto the Discrete Zero-Pole block inside.
      mask init: same as sensorMCU/Sensor Data/Raw Sensors/Sensor Suite/Low Pass6
      mask StyleString: edit,edit,edit,edit,edit,popup(zoh|foh|tustin|prewarp|matched),edit
      mask CallbackString: |||||hidecrit|
      mask Display:
      | droots(zeross,poless,gainss)
      | text( 0.5, 1.0, method, 'verticalAlignment','top')
  Low Pass3 : Subsystem  mask(DiscretizedZeroPole){Zeros=[], Poles=[-3], Gain=3, AbsTol=auto, SampleTime=T, method=tustin, Wc=1}
      mask prompts: Zeros "Zeros (enter in s-main:)"; Poles "Poles (enter in s-domain:)"; Gain "Gain (enter in s-domain:)"; AbsTol "Absolute tolerance:"; SampleTime "Sample time:"; Wc "Critical Frequency (Hz):"
      mask help: Continuous mask uses c2d to transform parameters onto the Discrete Zero-Pole block inside.
      mask init: same as sensorMCU/Sensor Data/Raw Sensors/Sensor Suite/Low Pass6
      mask StyleString: edit,edit,edit,edit,edit,popup(zoh|foh|tustin|prewarp|matched),edit
      mask CallbackString: |||||hidecrit|
      mask Display:
      | droots(zeross,poless,gainss)
      | text( 0.5, 1.0, method, 'verticalAlignment','top')
  Low Pass8 : Subsystem  mask(DiscretizedZeroPole){Zeros=[], Poles=[-3], Gain=3, AbsTol=auto, SampleTime=T, method=tustin, Wc=1}
      mask prompts: Zeros "Zeros (enter in s-main:)"; Poles "Poles (enter in s-domain:)"; Gain "Gain (enter in s-domain:)"; AbsTol "Absolute tolerance:"; SampleTime "Sample time:"; Wc "Critical Frequency (Hz):"
      mask help: Continuous mask uses c2d to transform parameters onto the Discrete Zero-Pole block inside.
      mask init: same as sensorMCU/Sensor Data/Raw Sensors/Sensor Suite/Low Pass6
      mask StyleString: edit,edit,edit,edit,edit,popup(zoh|foh|tustin|prewarp|matched),edit
      mask CallbackString: |||||hidecrit|
      mask Display:
      | droots(zeross,poless,gainss)
      | text( 0.5, 1.0, method, 'verticalAlignment','top')
  myMux Fun1 : Stateflow chart
  Temp Ini : Outport
  Gyro Ini Bias : Outport  Port=2
  wires:
  Temp Raw/1 -> Low Pass8/1(In1)
  Low Pass8/1(Out1) -> Temp Ini/1
  Gyro Raw/1 -> Demux/1
  Demux/1 -> Low Pass1/1(In1)
  Demux/2 -> Low Pass2/1(In1)
  Demux/3 -> Low Pass3/1(In1)
  Low Pass1/1(Out1) -> myMux Fun1/1(u1)
  Low Pass2/1(Out1) -> myMux Fun1/2(u2)
  Low Pass3/1(Out1) -> myMux Fun1/3(u3)
  myMux Fun1/1(y) -> Gyro Ini Bias/1

== system sensorMCU/Sensor Data/Raw Sensors/Sensor Suite/Calibration and Temperature Compensation/Mag Convert ==
  Raw : Inport
  Bias : Constant  Value=bias
  Divide : Product  Inputs=/*  OutScaling=2^-10
  Gains : Constant  Value=gains
  Sum : Sum  Inputs=|+-
  Comp : Outport
  wires:
  Bias/1 -> Sum/2
  Gains/1 -> Divide/1
  Sum/1 -> Divide/2
  Divide/1 -> Comp/1
  Raw/1 -> Sum/1

== system sensorMCU/Sensor Data/Raw Sensors/Sensor Suite/Calibration and Temperature Compensation/Mag Temp  Compensation ==
  Temp Raw : Inport
  Raw : Inport  Port=2
  Divide1 : Product  OutScaling=2^-10
  Mean Temperature for Calibration : Constant  Value=tempMean
  Sum1 : Sum  Inputs=|+-
  Sum2 : Sum  Inputs=|+-
  gains : Constant  Value=alpha
  Comp : Outport
  wires:
  Sum2/1 -> Comp/1
  Divide1/1 -> Sum2/2
  gains/1 -> Divide1/1
  Sum1/1 -> Divide1/2
  Temp Raw/1 -> Sum1/1
  Raw/1 -> Sum2/1
  Mean Temperature for Calibration/1 -> Sum1/2

== system sensorMCU/Sensor Data/Raw Sensors/Sensor Suite/Magnetometer Driver and Low Pass/Low Pass3 ==
  In1 : Inport
  Discrete Zero-Pole : DiscreteZeroPole  Zeros=zerosd  Poles=polesd  Gain=gaind  SampleTime=SampleTime
  Out1 : Outport
  wires:
  In1/1 -> Discrete Zero-Pole/1
  Discrete Zero-Pole/1 -> Out1/1

== system sensorMCU/Sensor Data/Raw Sensors/Sensor Suite/Magnetometer Driver and Low Pass/Low Pass4 ==
  In1 : Inport
  Discrete Zero-Pole : DiscreteZeroPole  Zeros=zerosd  Poles=polesd  Gain=gaind  SampleTime=SampleTime
  Out1 : Outport
  wires:
  Discrete Zero-Pole/1 -> Out1/1
  In1/1 -> Discrete Zero-Pole/1

== system sensorMCU/Sensor Data/Raw Sensors/Sensor Suite/Magnetometer Driver and Low Pass/Low Pass5 ==
  In1 : Inport
  Discrete Zero-Pole : DiscreteZeroPole  Zeros=zerosd  Poles=polesd  Gain=gaind  SampleTime=SampleTime
  Out1 : Outport
  wires:
  In1/1 -> Discrete Zero-Pole/1
  Discrete Zero-Pole/1 -> Out1/1

== system sensorMCU/Sensor Data/Raw Sensors/Sensor Suite/Subsystem/BaroConvert ==
  "Baro, raw" : Inport
  Gain : Gain  Gain=gains
  Sum1 : Sum  Inputs=|++
  bias : Constant  Value=bias
  Baro (Pa) : Outport
  wires:
  "Baro, raw"/1 -> Gain/1
  Sum1/1 -> Baro (Pa)/1
  Gain/1 -> Sum1/1
  bias/1 -> Sum1/2

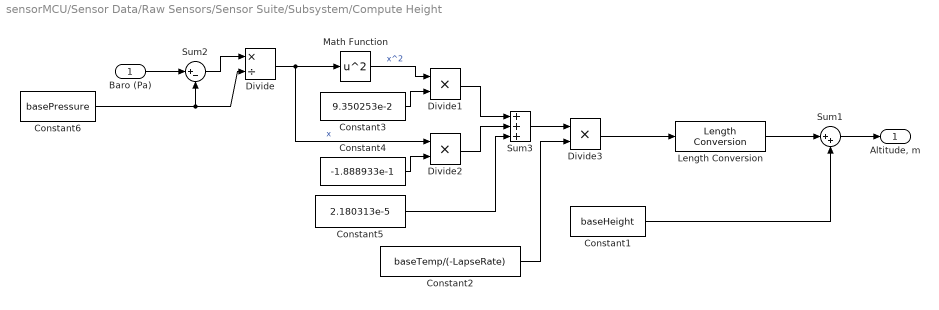
== system sensorMCU/Sensor Data/Raw Sensors/Sensor Suite/Subsystem/Compute Height ==
  Baro (Pa) : Inport
  Constant1 : Constant  Value=baseHeight
  Constant2 : Constant  Value=baseTemp/(-LapseRate)
  Constant3 : Constant  Value=9.350253e-2
  Constant4 : Constant  Value=-1.888933e-1
  Constant5 : Constant  Value=2.180313e-5
  Constant6 : Constant  Value=basePressure
  Divide : Product  Inputs=*/  OutScaling=2^-10
  Divide1 : Product  OutScaling=2^-10
  Divide2 : Product  OutScaling=2^-10
  Divide3 : Product  OutScaling=2^-10
  Length Conversion : aerolibconvert2/Length Conversion  SystemSampleTime=-1  IU=ft  OU=m
  Math Function : Math  Operator=square  SaturateOnIntegerOverflow=on
  Sum1 : Sum  Inputs=|++
  Sum2 : Sum  Inputs=|+-
  Sum3 : Sum  Inputs=3
  "Altitude, m" : Outport
  wires:
  Length Conversion/1 -> Sum1/1
  Sum2/1 -> Divide/1
  Sum1/1 -> "Altitude, m"/1
  Divide3/1 -> Length Conversion/1
  Constant2/1 -> Divide3/2
  Sum3/1 -> Divide3/1
  Constant5/1 -> Sum3/3
  Divide2/1 -> Sum3/2
  Divide1/1 -> Sum3/1
  Constant4/1 -> Divide2/2
  Constant3/1 -> Divide1/2
  Math Function/1 -> Divide1/1  "x^2"
  Divide/1 -> Divide2/1, Math Function/1  "x"
  Constant6/1 -> Divide/2, Sum2/2
  Constant1/1 -> Sum1/2
  Baro (Pa)/1 -> Sum2/1

== system sensorMCU/Sensor Data/Raw Sensors/Sensor Suite/Subsystem/Low Pass1 ==
  In1 : Inport
  Discrete Zero-Pole : DiscreteZeroPole  Zeros=zerosd  Poles=polesd  Gain=gaind  SampleTime=SampleTime
  Out1 : Outport
  wires:
  In1/1 -> Discrete Zero-Pole/1
  Discrete Zero-Pole/1 -> Out1/1

== system sensorMCU/Sensor Data/Raw Sensors/Sensor Suite/Subsystem/Low Pass10 ==
  In1 : Inport
  Discrete Zero-Pole : DiscreteZeroPole  Zeros=zerosd  Poles=polesd  Gain=gaind  SampleTime=SampleTime
  Out1 : Outport
  wires:
  In1/1 -> Discrete Zero-Pole/1
  Discrete Zero-Pole/1 -> Out1/1

== system sensorMCU/Sensor Data/Raw Sensors/Sensor Suite/Subsystem/Low Pass2 ==
  In1 : Inport
  Discrete Zero-Pole : DiscreteZeroPole  Zeros=zerosd  Poles=polesd  Gain=gaind  SampleTime=SampleTime
  Out1 : Outport
  wires:
  Discrete Zero-Pole/1 -> Out1/1
  In1/1 -> Discrete Zero-Pole/1

== system sensorMCU/Sensor Data/Raw Sensors/Sensor Suite/Subsystem/Low Pass8 ==
  In1 : Inport
  Discrete Zero-Pole : DiscreteZeroPole  Zeros=zerosd  Poles=polesd  Gain=gaind  SampleTime=SampleTime
  Out1 : Outport
  wires:
  In1/1 -> Discrete Zero-Pole/1
  Discrete Zero-Pole/1 -> Out1/1

== system sensorMCU/Sensor Data/Raw Sensors/Sensor Suite/Subsystem/Mag Temp  Compensation1 ==
  Raw : Inport
  Temp Raw : Inport  Port=2
  Divide1 : Product  OutScaling=2^-10
  Mean Temperature for Calibration : Constant  Value=tempMean
  Sum1 : Sum  Inputs=|+-
  Sum2 : Sum  Inputs=|+-
  gains : Constant  Value=alpha
  Comp : Outport
  wires:
  Mean Temperature for Calibration/1 -> Sum1/2
  Raw/1 -> Sum2/1
  Temp Raw/1 -> Sum1/1
  Sum1/1 -> Divide1/2
  gains/1 -> Divide1/1
  Divide1/1 -> Sum2/2
  Sum2/1 -> Comp/1

== system sensorMCU/Position-Attitude Filter/GPS parser/Geod2LTP2/ECEF2LTP (UEN)/From Body to Universal1/Rotation Matrix from Long//Lat ==
  note: Calculate Coefficients of DCM Row-Wise
  long lat : Inport
  11 : Fcn  Expr=cos(u[1])*cos(u[2])
  12 : Fcn  Expr=sin(u[1])*cos(u[2])
  13 : Fcn  Expr=sin(u[2])
  21 : Fcn  Expr=-sin(u[1])
  22 : Fcn  Expr=cos(u[1])
  23 : Fcn  Expr=0
  31 : Fcn  Expr=-sin(u[2])*cos(u[1])
  32 : Fcn  Expr=-sin(u[1])*sin(u[2])
  33 : Fcn  Expr=cos(u[2])
  Mux2 : Mux  Inputs=9
  DCM : Outport  InitialOutput=0
  wires:
  33/1 -> Mux2/9
  23/1 -> Mux2/8
  13/1 -> Mux2/7
  32/1 -> Mux2/6
  22/1 -> Mux2/5
  12/1 -> Mux2/4
  31/1 -> Mux2/3
  21/1 -> Mux2/2
  11/1 -> Mux2/1
  Mux2/1 -> DCM/1
  long lat/1 -> 11/1, 33/1, 23/1, 13/1, 32/1, 22/1, 12/1, 31/1, 21/1

== system sensorMCU/Sensor Data/Raw Sensors/Sensor Suite/Calibration and Temperature Compensation/Initial Bias and Temp/Low Pass1 ==
  In1 : Inport
  Discrete Zero-Pole : DiscreteZeroPole  Zeros=zerosd  Poles=polesd  Gain=gaind  SampleTime=SampleTime
  Out1 : Outport
  wires:
  Discrete Zero-Pole/1 -> Out1/1
  In1/1 -> Discrete Zero-Pole/1

== system sensorMCU/Sensor Data/Raw Sensors/Sensor Suite/Calibration and Temperature Compensation/Initial Bias and Temp/Low Pass2 ==
  In1 : Inport
  Discrete Zero-Pole : DiscreteZeroPole  Zeros=zerosd  Poles=polesd  Gain=gaind  SampleTime=SampleTime
  Out1 : Outport
  wires:
  In1/1 -> Discrete Zero-Pole/1
  Discrete Zero-Pole/1 -> Out1/1

== system sensorMCU/Sensor Data/Raw Sensors/Sensor Suite/Calibration and Temperature Compensation/Initial Bias and Temp/Low Pass3 ==
  In1 : Inport
  Discrete Zero-Pole : DiscreteZeroPole  Zeros=zerosd  Poles=polesd  Gain=gaind  SampleTime=SampleTime
  Out1 : Outport
  wires:
  Discrete Zero-Pole/1 -> Out1/1
  In1/1 -> Discrete Zero-Pole/1

== system sensorMCU/Sensor Data/Raw Sensors/Sensor Suite/Calibration and Temperature Compensation/Initial Bias and Temp/Low Pass8 ==
  In1 : Inport
  Discrete Zero-Pole : DiscreteZeroPole  Zeros=zerosd  Poles=polesd  Gain=gaind  SampleTime=SampleTime
  Out1 : Outport
  wires:
  In1/1 -> Discrete Zero-Pole/1
  Discrete Zero-Pole/1 -> Out1/1

== matlab function Sensor Data/Raw Sensors/Sensor Suite/Magnetometer Driver and Low Pass/Magnetometer Driver ==
  data: mag_k output inherited; M_in input inherited
function mag_k  = M_out(M_in)
% This is the Magnetometer driver

    persistent M_old;
    persistent clk;
    persistent magOld;
    persistent cycCount; 
    persistent zSign; 
    sampDif  =0;
    rnMax = 0;
    
    if isempty(M_old)
        M_old = [0; 0; 0];
        clk = 1;
        magOld = [0; 0 ; 0];
        cycCount =0;
        zSign =1;
    end
    
    if cycCount  < 50
        cycCount = cycCount + 1;
    end

    %rnMax = find (M_in == max(M_in));
    % Code replacement for find function (not supported in EML)
    if M_in(1) > M_in(2)
        if M_in(1)> M_in(3)
            rnMax = 1;
        else
            rnMax = 3;
        end
    else
        if M_in(2)>M_in(3)
            rnMax = 2;
        else
            rnMax = 3;
        end;
    end
    
    sampDif =  M_in(rnMax(1))- M_old(rnMax(1));
    
    if ~(sampDif > -15 && sampDif < 15)
        clk = -clk;
        mag_k = clk*(M_in-M_old).*0.5;
    else
        mag_k = magOld.*[1 1 zSign]';
    end;
    
    if cycCount == 50
        if mag_k(3)> 0
            zSign = -1;
        end
        cycCount = cycCount +1;
    end
    
    mag_k(3)= zSign*mag_k(3);
    M_old = M_in;
    magOld = mag_k;
end

== matlab function To Control MCU/myMux Fun ==
  data: u1 input inherited; y output inherited; u2 input inherited; u3 input inherited; u4 input inherited; u5 input inherited; u6 input inherited; u7 input inherited; u8 input inherited; u9 input inherited; u10 input inherited
function y = myMux(u1, u2, u3, u4, u5, u6, u7, u8, u9, u10)
% This block supports an embeddable subset of the MATLAB language.
% See the help menu for details. 

y = [u1(:); u2(:); u3(:); u4(:); u5(:); u6(:); u7(:); u8(:); u9(1); u10(:)];
